simulink library "sensors"  (R2025b)
settings: Solver=VariableStepAuto  StartTime=0.0  StopTime=10.0  RelTol=1e-3
undefined symbols (not defined in the file or in its folder): D_bias_inst, D_RW, DiscIntNeverNeededParam, sens_eh_bias_instability, sens_eh_bias_pitch, sens_eh_bias_roll, sens_eh_C_misalign, sens_eh_noise_power, sens_eh_scale_factor_error, sens_eh_Ts, sens_gyro, sens_gyro_D_bias_inst, sens_gyro_D_RW, sens_gyro_D_wn, sens_gyro_O, sens_gyro_run_run_bias, sens_gyro_SFE, sens_gyro_SFN, sens_gyro_static_temp_bias, sens_gyro_theta_eps, sens_gyro_Ts, Ts_gyro
libraries: simulink_extras x4
settings Model: Creator=nicol  LastModifiedBy=nicol

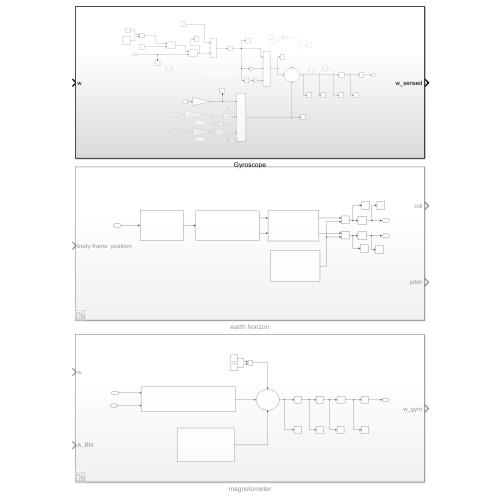
[thumbnail: Simulink's stored preview of the top-level diagram]
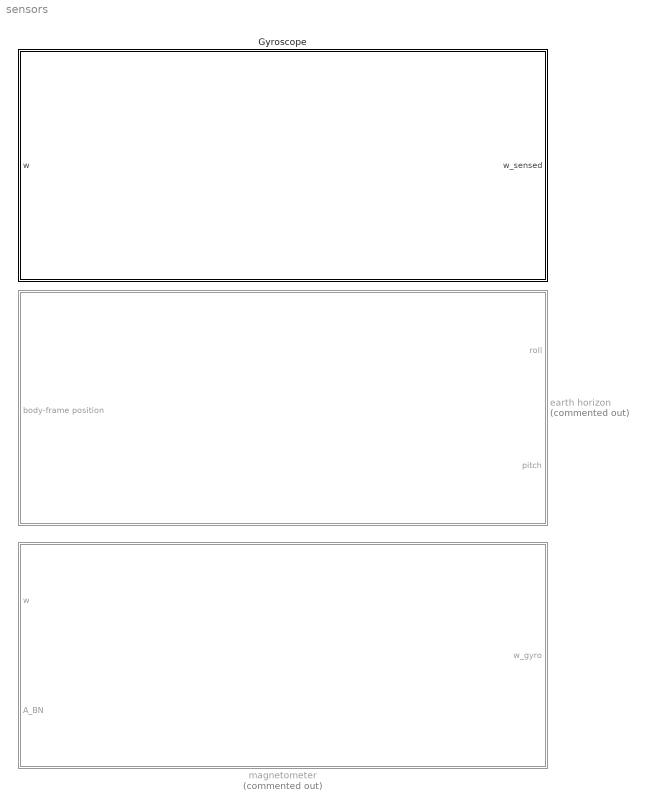
== system sensors ==
  Gyroscope : Subsystem
  earth horizon : Subsystem  Commented=on
  magnetometer : Subsystem  Commented=on

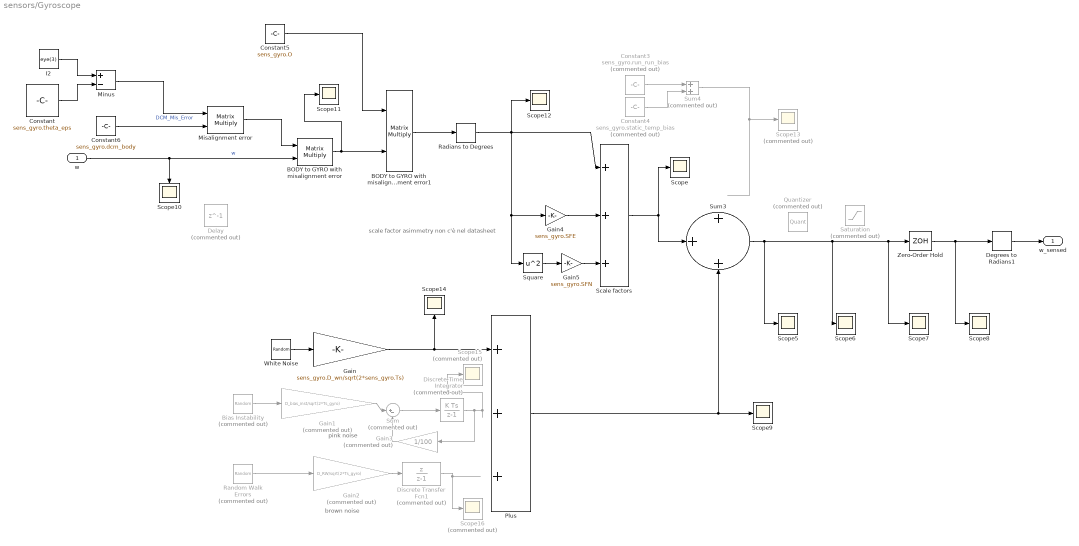
== system sensors/Gyroscope ==
  note: pink noise
  note: brown noise
  note: scale factor asimmetry non c'è nel datasheet
  w : Inport
  " White Noise" : RandomNumber  SampleTime=sens_gyro.Ts
  BODY to GYRO with misalignment error : Product  Multiplication=Matrix(*)
  BODY to GYRO with misalignment error1 : Product  Multiplication=Matrix(*)
  Bias Instability : RandomNumber  Commented=on  SampleTime=Ts_gyro
  Constant : Constant  Value=sens_gyro.theta_eps
  Constant3 : Constant  Commented=on  Value=sens_gyro.run_run_bias
  Constant4 : Constant  Commented=on  Value=sens_gyro.static_temp_bias
  Constant5 : Constant  Value=sens_gyro.O
  Constant6 : Constant  Value=sens_gyro.dcm_body
  Degrees to Radians1 : simulink_extras/Transformations/Degrees to Radians
  Delay : Delay  Commented=on  DelayLength=1  SampleTime=sens_gyro_Ts
  Discrete Transfer Fcn1 : DiscreteTransferFcn  Commented=on  Numerator=[1 0]  Denominator=[1 -1]
  Discrete-Time Integrator : DiscreteIntegrator  Commented=on  SampleTime=Ts_gyro  ICPrevOutput=DiscIntNeverNeededParam  ICPrevScaledInput=DiscIntNeverNeededParam
  Gain : Gain  Gain=sens_gyro.D_wn/sqrt(2*sens_gyro.Ts)
  Gain1 : Gain  Commented=on  Gain=D_bias_inst/sqrt(2*Ts_gyro)
  Gain2 : Gain  Commented=on  Gain=D_RW/sqrt(2*Ts_gyro)
  Gain3 : Gain  Commented=on  Gain=1/100
  Gain4 : Gain  Gain=sens_gyro.SFE
  Gain5 : Gain  Gain=sens_gyro.SFN
  I2 : Constant  Value=eye(3)
  Minus : Sum  Inputs=+-
  Misalignment error : Product  Multiplication=Matrix(*)
  Plus : Sum  Inputs=+++
  Quantizer : Quantizer  Commented=on  QuantizationInterval=sens_gyro.LSB
  Radians to Degrees : simulink_extras/Transformations/Radians to Degrees
  Random Walk Errors : RandomNumber  Commented=on  SampleTime=Ts_gyro
  Saturation : Saturate  Commented=on  UpperLimit=20  LowerLimit=-20
  Scale factors : Sum  Inputs=+++
  Scope{,5..12,14} (10 alike) : Scope
      Scope settings: ActiveDisplayYMinimum=-0.05312900609083622  ActiveDisplayYMaximum=0.12066272542819415  DataLoggingVariableName=ScopeData21
      Scope10 settings: ActiveDisplayYMinimum=-0.00056894172246074542  ActiveDisplayYMaximum=0.0021576003098755735  DataLoggingVariableName=ScopeData18
      Scope11 settings: ActiveDisplayYMinimum=-0.00092681479365303444  ActiveDisplayYMaximum=0.0021049073575945929  DataLoggingVariableName=ScopeData19
      Scope12 settings: ActiveDisplayYMinimum=-0.053102456426698724  ActiveDisplayYMaximum=0.12060224686521961  DataLoggingVariableName=ScopeData20
      Scope14 settings: ActiveDisplayYMinimum=-0.0017013348354620785  ActiveDisplayYMaximum=0.001720930099973718  DataLoggingVariableName=ScopeData23
      Scope5 settings: ActiveDisplayYMinimum=-0.50665069153891817  ActiveDisplayYMaximum=0.44875689729546858  DataLoggingVariableName=ScopeData26
      Scope6 settings: ActiveDisplayYMinimum=-0.084211031923642515  ActiveDisplayYMaximum=0.1503467797108943  DataLoggingVariableName=ScopeData27
      Scope7 settings: ActiveDisplayYMinimum=-0.056158896455048  ActiveDisplayYMaximum=0.14157783649801767  DataLoggingVariableName=ScopeData28
      Scope8 settings: ActiveDisplayYMinimum=-0.4247782676928904  ActiveDisplayYMaximum=0.16214242495577319  DataLoggingVariableName=ScopeData29
      Scope9 settings: ActiveDisplayYMinimum=-0.028049471714822149  ActiveDisplayYMaximum=0.023551833456329586  DataLoggingVariableName=ScopeData30
  Scope13 : Scope  Commented=on
      settings: ActiveDisplayYMinimum=0.0021581201979827048  ActiveDisplayYMaximum=0.0049044990082149995  DataLoggingVariableName=ScopeData22
  Scope15 : Scope  Commented=on
      settings: ActiveDisplayYMinimum=-0.0014348986053723438  ActiveDisplayYMaximum=0.0031607957597654607  DataLoggingVariableName=ScopeData24
  Scope16 : Scope  Commented=on
      settings: ActiveDisplayYMinimum=-0.025854146894594331  ActiveDisplayYMaximum=0.0028201702031084522  DataLoggingVariableName=ScopeData25
  Square : Math  Operator=square
  Sum : Sum  Commented=on  Inputs=|+-
  Sum3 : Sum  Inputs=+++
  Sum4 : Sum  Commented=on
  Zero-Order Hold : ZeroOrderHold  SampleTime=sens_gyro.Ts
  w_sensed : Outport
  wires:
  Misalignment error/1 -> BODY to GYRO with misalignment error/1
  Degrees to Radians1/1 -> w_sensed/1
  BODY to GYRO with misalignment error/1 -> Scope11/1, BODY to GYRO with misalignment error1/2
  Constant6/1 -> Misalignment error/2
  Constant4/1 -> Sum4/2
  Discrete-Time Integrator/1 -> Gain3/1, Scope15/1
  Sum/1 -> Discrete-Time Integrator/1
  Random Walk Errors/1 -> Gain2/1
  Sum3/1 -> Scope7/1, Zero-Order Hold/1, Scope6/1, Scope5/1
  Discrete Transfer Fcn1/1 -> Scope16/1
  Scale factors/1 -> Sum3/2, Scope/1
  I2/1 -> Minus/1
  Minus/1 -> Misalignment error/1  "DCM_Mis_Error"
  Zero-Order Hold/1 -> Degrees to Radians1/1, Scope8/1
  Gain5/1 -> Scale factors/3
  Gain1/1 -> Sum/1
  Radians to Degrees/1 -> Scope12/1, Gain4/1, Square/1, Scale factors/1
  Constant5/1 -> BODY to GYRO with misalignment error1/1
  " White Noise"/1 -> Gain/1
  Square/1 -> Gain5/1
  Bias Instability/1 -> Gain1/1
  Sum4/1 -> Scope13/1
  w/1 -> BODY to GYRO with misalignment error/2, Scope10/1  "w"
  Gain/1 -> Scope14/1, Plus/1
  Constant3/1 -> Sum4/1
  Constant/1 -> Minus/2
  BODY to GYRO with misalignment error1/1 -> Radians to Degrees/1
  Gain3/1 -> Sum/2
  Gain4/1 -> Scale factors/2
  Gain2/1 -> Discrete Transfer Fcn1/1
  Plus/1 -> Sum3/3, Scope9/1

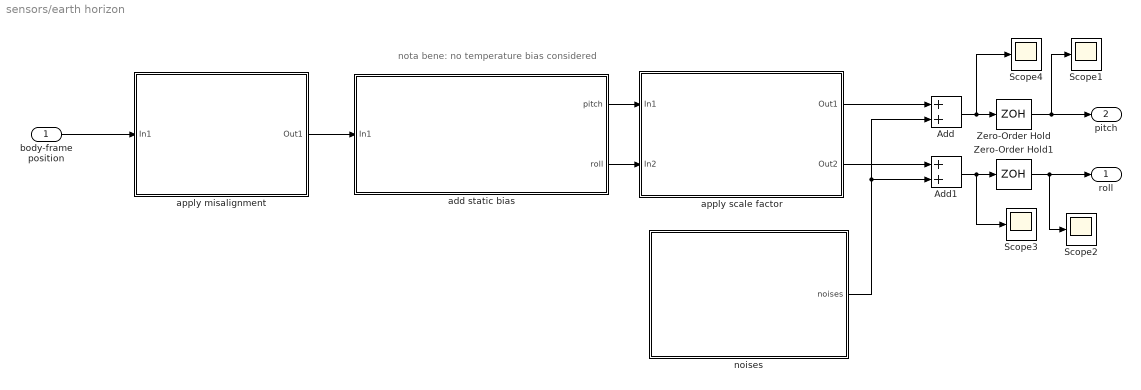
== system sensors/earth horizon ==
  note: nota bene: no temperature bias considered
  body-frame position : Inport
  Add : Sum
  Add1 : Sum
  Scope{1..4} (4 alike) : Scope
      Scope1 settings: ActiveDisplayYMinimum=1.5625791702895984  ActiveDisplayYMaximum=1.6764041605673214  DataLoggingVariableName=ScopeData6
      Scope2 settings: ActiveDisplayYMinimum=-1  ActiveDisplayYMaximum=1  DataLoggingVariableName=ScopeData7
      Scope3 settings: ActiveDisplayYMinimum=-1  ActiveDisplayYMaximum=1  DataLoggingVariableName=ScopeData10
      Scope4 settings: ActiveDisplayYMinimum=1.4889132362766662  ActiveDisplayYMaximum=1.7377766761477982  DataLoggingVariableName=ScopeData9
  Zero-Order Hold : ZeroOrderHold  SampleTime=sens_eh_Ts
  Zero-Order Hold1 : ZeroOrderHold  SampleTime=sens_eh_Ts
  add static bias : Subsystem
  apply misalignment : Subsystem
  apply scale factor : Subsystem
  noises : Subsystem
  roll : Outport
  pitch : Outport  Port=2
  wires:
  body-frame position/1 -> apply misalignment/1(In1)
  Zero-Order Hold/1 -> Scope1/1, pitch/1
  apply misalignment/1(Out1) -> add static bias/1(In1)
  noises/1(noises) -> Add1/2, Add/2
  apply scale factor/2(Out2) -> Add1/1
  apply scale factor/1(Out1) -> Add/1
  Add/1 -> Zero-Order Hold/1, Scope4/1
  Add1/1 -> Zero-Order Hold1/1, Scope3/1
  Zero-Order Hold1/1 -> Scope2/1, roll/1
  add static bias/2(roll) -> apply scale factor/2(In2)
  add static bias/1(pitch) -> apply scale factor/1(In1)

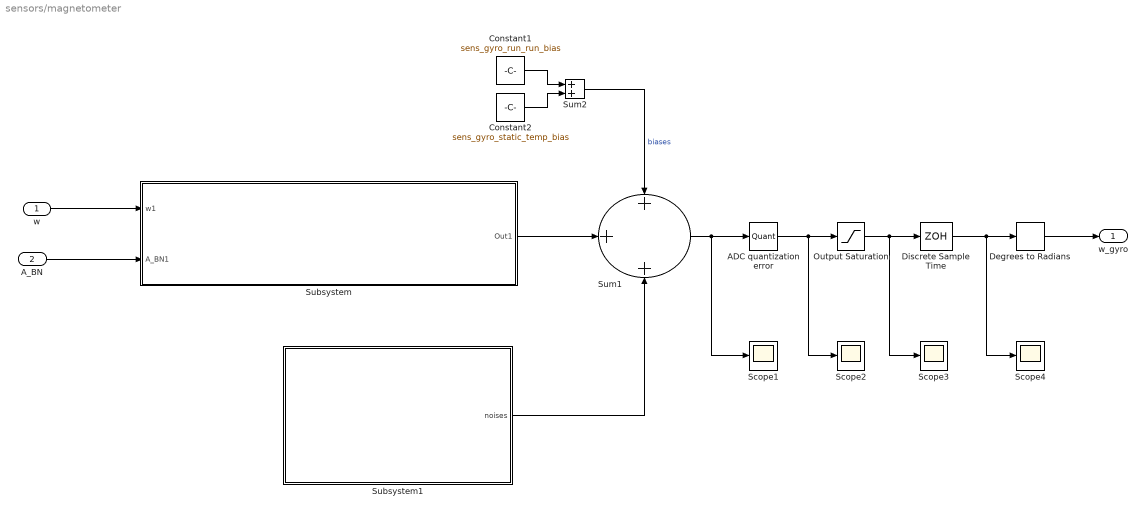
== system sensors/magnetometer ==
  w : Inport
  A_BN : Inport  Port=2
  ADC quantization error : Quantizer  QuantizationInterval=sens_gyro_LSB
  Constant1 : Constant  Value=sens_gyro_run_run_bias
  Constant2 : Constant  Value=sens_gyro_static_temp_bias
  Degrees to Radians : simulink_extras/Transformations/Degrees to Radians
  Discrete Sample Time : ZeroOrderHold  SampleTime=sens_gyro_Ts
  Output Saturation : Saturate  UpperLimit=20  LowerLimit=-20
  Scope{1..4} (4 alike) : Scope
      Scope1 settings: ActiveDisplayYMinimum=-0.032120647567430112  ActiveDisplayYMaximum=0.096644162809020939  DataLoggingVariableName=ScopeData14
      Scope2 settings: ActiveDisplayYMinimum=-1  ActiveDisplayYMaximum=1  DataLoggingVariableName=ScopeData15
      Scope3 settings: ActiveDisplayYMinimum=-1  ActiveDisplayYMaximum=1  DataLoggingVariableName=ScopeData16
      Scope4 settings: ActiveDisplayYMinimum=-0.032120647471039  ActiveDisplayYMaximum=0.096644162883216228  DataLoggingVariableName=ScopeData17
  Subsystem : Subsystem
  Subsystem1 : Subsystem
  Sum1 : Sum  Inputs=+++
  Sum2 : Sum
  w_gyro : Outport
  wires:
  Constant2/1 -> Sum2/2
  Subsystem1/1(noises) -> Sum1/3
  Subsystem/1(Out1) -> Sum1/2
  ADC quantization error/1 -> Output Saturation/1, Scope2/1
  Sum1/1 -> ADC quantization error/1, Scope1/1
  Discrete Sample Time/1 -> Degrees to Radians/1, Scope4/1
  Sum2/1 -> Sum1/1  "biases"
  w/1 -> Subsystem/1(w1)
  Degrees to Radians/1 -> w_gyro/1
  Constant1/1 -> Sum2/1
  A_BN/1 -> Subsystem/2(A_BN1)
  Output Saturation/1 -> Discrete Sample Time/1, Scope3/1

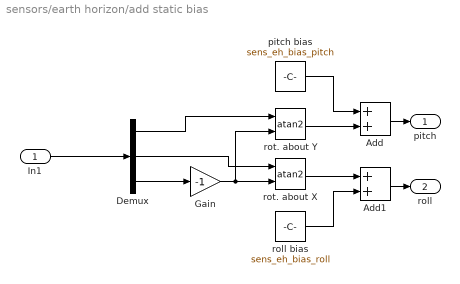
== system sensors/earth horizon/add static bias ==
  In1 : Inport
  Add : Sum
  Add1 : Sum
  Demux : Demux  Outputs=3
  Gain : Gain  Gain=-1
  pitch bias : Constant  Value=sens_eh_bias_pitch
  roll bias : Constant  Value=sens_eh_bias_roll
  rot. about X : Trigonometry  Operator=atan2
  rot. about Y : Trigonometry  Operator=atan2
  pitch : Outport
  roll : Outport  Port=2
  wires:
  In1/1 -> Demux/1
  Add/1 -> pitch/1
  Add1/1 -> roll/1
  Demux/3 -> Gain/1
  pitch bias/1 -> Add/1
  Demux/1 -> rot. about Y/1
  Demux/2 -> rot. about X/1
  rot. about Y/1 -> Add/2
  rot. about X/1 -> Add1/1
  Gain/1 -> rot. about Y/2, rot. about X/2
  roll bias/1 -> Add1/2

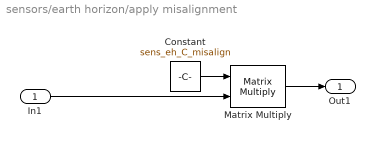
== system sensors/earth horizon/apply misalignment ==
  In1 : Inport
  Constant : Constant  Value=sens_eh_C_misalign
  Matrix Multiply : Product  Multiplication=Matrix(*)
  Out1 : Outport
  wires:
  Matrix Multiply/1 -> Out1/1
  Constant/1 -> Matrix Multiply/1
  In1/1 -> Matrix Multiply/2

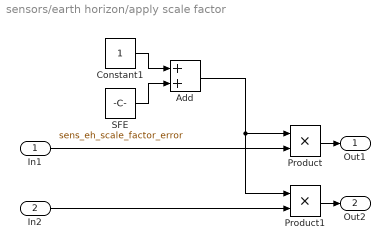
== system sensors/earth horizon/apply scale factor ==
  In1 : Inport
  In2 : Inport  Port=2
  Add : Sum
  Constant1 : Constant
  Product : Product
  Product1 : Product
  SFE : Constant  Value=sens_eh_scale_factor_error
  Out1 : Outport
  Out2 : Outport  Port=2
  wires:
  Product/1 -> Out1/1
  Constant1/1 -> Add/1
  In2/1 -> Product1/2
  SFE/1 -> Add/2
  Product1/1 -> Out2/1
  Add/1 -> Product/1, Product1/1
  In1/1 -> Product/2

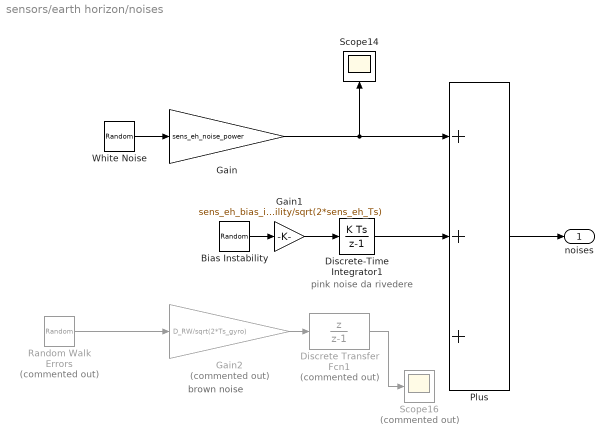
== system sensors/earth horizon/noises ==
  note: pink noise da rivedere
  note: brown noise
  " White Noise" : RandomNumber  SampleTime=sens_eh_Ts
  Bias Instability : RandomNumber  SampleTime=sens_eh_Ts
  Discrete Transfer Fcn1 : DiscreteTransferFcn  Commented=on  Numerator=[1 0]  Denominator=[1 -1]
  Discrete-Time Integrator1 : DiscreteIntegrator  SampleTime=sens_eh_Ts  ICPrevOutput=DiscIntNeverNeededParam  ICPrevScaledInput=DiscIntNeverNeededParam
  Gain : Gain  Gain=sens_eh_noise_power
  Gain1 : Gain  Gain=sens_eh_bias_instability/sqrt(2*sens_eh_Ts)
  Gain2 : Gain  Commented=on  Gain=D_RW/sqrt(2*Ts_gyro)
  Plus : Sum  Inputs=+++
  Random Walk Errors : RandomNumber  Commented=on  SampleTime=Ts_gyro
  Scope14 : Scope
      settings: ActiveDisplayYMinimum=-0.0017013348354620785  ActiveDisplayYMaximum=0.001720930099973718  DataLoggingVariableName=ScopeData23
  Scope16 : Scope  Commented=on
      settings: ActiveDisplayYMinimum=-0.025854146894594331  ActiveDisplayYMaximum=0.0028201702031084522  DataLoggingVariableName=ScopeData25
  noises : Outport
  wires:
  Bias Instability/1 -> Gain1/1
  Discrete-Time Integrator1/1 -> Plus/2
  Gain1/1 -> Discrete-Time Integrator1/1
  Gain2/1 -> Discrete Transfer Fcn1/1
  " White Noise"/1 -> Gain/1
  Random Walk Errors/1 -> Gain2/1
  Gain/1 -> Scope14/1, Plus/1
  Discrete Transfer Fcn1/1 -> Scope16/1
  Plus/1 -> noises/1

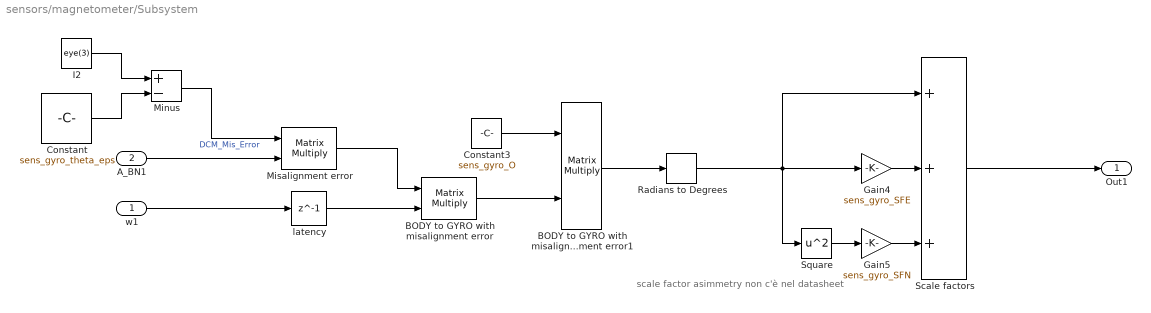
== system sensors/magnetometer/Subsystem ==
  note: scale factor asimmetry non c'è nel datasheet
  w1 : Inport
  A_BN1 : Inport  Port=2
  BODY to GYRO with misalignment error : Product  Multiplication=Matrix(*)
  BODY to GYRO with misalignment error1 : Product  Multiplication=Matrix(*)
  Constant : Constant  Value=sens_gyro_theta_eps
  Constant3 : Constant  Value=sens_gyro_O
  Gain4 : Gain  Gain=sens_gyro_SFE
  Gain5 : Gain  Gain=sens_gyro_SFN
  I2 : Constant  Value=eye(3)
  Minus : Sum  Inputs=+-
  Misalignment error : Product  Multiplication=Matrix(*)
  Radians to Degrees : simulink_extras/Transformations/Radians to Degrees
  Scale factors : Sum  Inputs=+++
  Square : Math  Operator=square
  latency : Delay  DelayLength=1
  Out1 : Outport
  wires:
  Constant/1 -> Minus/2
  w1/1 -> latency/1
  Constant3/1 -> BODY to GYRO with misalignment error1/1
  Gain4/1 -> Scale factors/2
  A_BN1/1 -> Misalignment error/2
  Radians to Degrees/1 -> Square/1, Gain4/1, Scale factors/1
  Gain5/1 -> Scale factors/3
  BODY to GYRO with misalignment error1/1 -> Radians to Degrees/1
  Square/1 -> Gain5/1
  Misalignment error/1 -> BODY to GYRO with misalignment error/1
  latency/1 -> BODY to GYRO with misalignment error/2
  I2/1 -> Minus/1
  BODY to GYRO with misalignment error/1 -> BODY to GYRO with misalignment error1/2
  Minus/1 -> Misalignment error/1  "DCM_Mis_Error"
  Scale factors/1 -> Out1/1

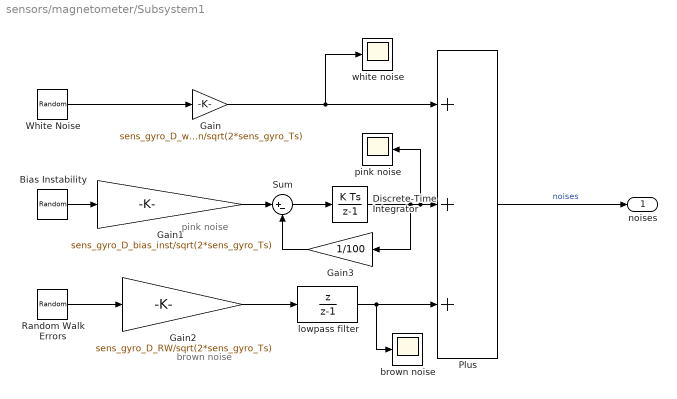
== system sensors/magnetometer/Subsystem1 ==
  note: pink noise
  note: brown noise
  " White Noise" : RandomNumber  SampleTime=0.1
  Bias Instability : RandomNumber  SampleTime=0.1
  Discrete-Time Integrator : DiscreteIntegrator  ICPrevOutput=DiscIntNeverNeededParam  ICPrevScaledInput=DiscIntNeverNeededParam
  Gain : Gain  Gain=sens_gyro_D_wn/sqrt(2*sens_gyro_Ts)
  Gain1 : Gain  Gain=sens_gyro_D_bias_inst/sqrt(2*sens_gyro_Ts)
  Gain2 : Gain  Gain=sens_gyro_D_RW/sqrt(2*sens_gyro_Ts)
  Gain3 : Gain  Gain=1/100
  Plus : Sum  Inputs=+++
  Random Walk Errors : RandomNumber  SampleTime=0.1
  Sum : Sum  Inputs=|+-
  brown noise : Scope
      settings: ActiveDisplayYMinimum=-0.025691906984189852  ActiveDisplayYMaximum=0.0025755592198982418  DataLoggingVariableName=ScopeData11
  lowpass filter : DiscreteTransferFcn  Numerator=[1 0]  Denominator=[1 -1]
  pink noise : Scope
      settings: ActiveDisplayYMinimum=-0.013777619312277414  ActiveDisplayYMaximum=0.014220901201123974  DataLoggingVariableName=ScopeData12
  white noise : Scope
      settings: ActiveDisplayYMinimum=-0.0017013348354620785  ActiveDisplayYMaximum=0.001720930099973718  DataLoggingVariableName=ScopeData13
  noises : Outport
  wires:
  Random Walk Errors/1 -> Gain2/1
  Gain1/1 -> Sum/1
  lowpass filter/1 -> brown noise/1, Plus/3
  Gain/1 -> Plus/1, white noise/1
  Plus/1 -> noises/1  "noises"
  Gain3/1 -> Sum/2
  Bias Instability/1 -> Gain1/1
  Gain2/1 -> lowpass filter/1
  Sum/1 -> Discrete-Time Integrator/1
  " White Noise"/1 -> Gain/1
  Discrete-Time Integrator/1 -> Gain3/1, Plus/2, pink noise/1
